simulink model "reactor_2izoterm"  (R2021a)
settings: Solver=VariableStepAuto  StartTime=0.0  StopTime=10.0  RelTol=1e-3
values from neighbouring files (symbols this model uses):
  ci = 10    [script.m]
  EdR = 49584/8.32    (= 5959.61538462)    [script.m]
  k0 = 34930800    [script.m]
  Kr = Tp/(T0int*Kp)    (= 35.3982300885)    [script.m]
  Ti = 38+273    (= 311)    [script.m]
  Tint = Tp    (= 0.78)    [script.m]
  V = 10    [script.m]
libraries: pid_lib x1
settings Model: Creator=Automatica  LastModifiedBy=Automatica

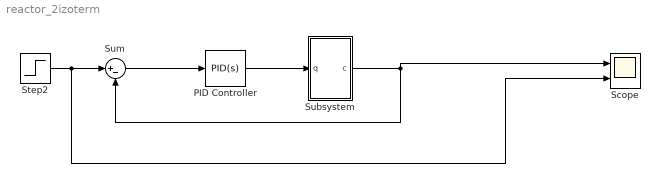
== system reactor_2izoterm ==
  PID Controller : pid_lib/PID Controller  Controller=PID  Form=Parallel  TimeDomain=Continuous-time  UseExternalTs=off  SampleTime=-1  IntegratorMethod=Forward Euler  FilterMethod=Forward Euler  ControllerParametersSource=internal  P=Kr  I=Kr/Tint  D=0  UseFilter=on  N=100  TunerSelectOption=Transfer Function Based (PID Tuner App)  InitialConditionSource=internal  InitialConditionForIntegrator=q  InitialConditionForFilter=0  DifferentiatorICPrevScaledInput=0  ExternalReset=none  TrackingMode=off  Kt=1  LimitOutput=off  SatLimitsSource=internal  UpperSaturationLimit=inf  LowerSaturationLimit=-inf  LinearizeAsGain=on  AntiWindupMode=none  Kb=1  POutMin=[]  POutMax=[]  IOutMin=[]  IOutMax=[]  DOutMin=[]  DOutMax=[]  NOutMin=[]  NOutMax=[]  SumOutMin=[]  SumOutMax=[]  SaturationOutMin=[]  SaturationOutMax=[]  PParamMin=[]  PParamMax=[]  IParamMin=[]  IParamMax=[]  DParamMin=[]  DParamMax=[]  NParamMin=[]  NParamMax=[]  KbParamMin=[]  KbParamMax=[]  KtParamMin=[]  KtParamMax=[]  KbOutMin=[]  KbOutMax=[]  KtOutMin=[]  KtOutMax=[]  IntegratorOutMin=[]  IntegratorOutMax=[]  FilterOutMin=[]  FilterOutMax=[]  SumI1OutMin=[]  SumI1OutMax=[]  SumI2OutMin=[]  SumI2OutMax=[]  SumI3OutMin=[]  SumI3OutMax=[]  SumI4OutMin=[]  SumI4OutMax=[]  SumDOutMin=[]  SumDOutMax=[]  DifferentiatorOutMin=[]  DifferentiatorOutMax=[]  FilterDiffOutCoefMin=[]  FilterDiffOutCoefMax=[]  ReciprocalOutMin=[]  ReciprocalOutMax=[]  SumDenOutMin=[]  SumDenOutMax=[]  SumNumOutMin=[]  SumNumOutMax=[]  DivideOutMin=[]  DivideOutMax=[]  UdiffTsProdOutMin=[]  UdiffTsProdOutMax=[]  NTsProdOutMin=[]  NTsProdOutMax=[]  UintegralTsProdOutMin=[]  UintegralTsProdOutMax=[]  UngainTsProdOutMin=[]  UngainTsProdOutMax=[]  IntegratorContinuousStateAttributes=''  IntegratorStateMustResolveToSignalObject=off  IntegratorRTWStateStorageClass=Auto  FilterContinuousStateAttributes=''  FilterStateMustResolveToSignalObject=off  FilterRTWStateStorageClass=Auto  ParallelPVariant=InternalParameters  IdealPVariant=Disabled  IVariant=InternalParameters  DVariant=InternalParameters  IntegratorVariant=Continuous  SatVariant=Disabled  AWVariant=Passthrough  PCopyVariant=Disabled  TRVariant=Disabled  FdbkBlocksVariant=Forward  IdealPFdbkVariant=Disabled  SatFdbkVariant=Disabled  DerivativeFilterVariant=ContFilter  NVariant=InternalParameters  NCopyVariant=Disabled  FilterICVariant=InternalICsFilter  IntegratorICVariant=InternalICs  ExternalResetVariant=Disabled  TRSumVariant=Passthrough  SumFdbkVariant=Disabled  SumVariant=Sum_PID  TsampFilterVariant=InternalTs  TsampNgainVariant=Passthrough  TsampIntegralVariant=Passthrough  ExternalSaturationOutDataTypeStr=Inherit: Same as second input
  Scope : Scope  NumInputPorts=2
  Step2 : Step  Time=0  Before=8.574  After=8.574+0.1  SampleTime=0
  Subsystem : Subsystem
  Sum : Sum  Inputs=|+-
  wires:
  Subsystem/1(c) -> Sum/2, Scope/1
  Step2/1 -> Scope/2, Sum/1
  PID Controller/1 -> Subsystem/1(q)
  Sum/1 -> PID Controller/1

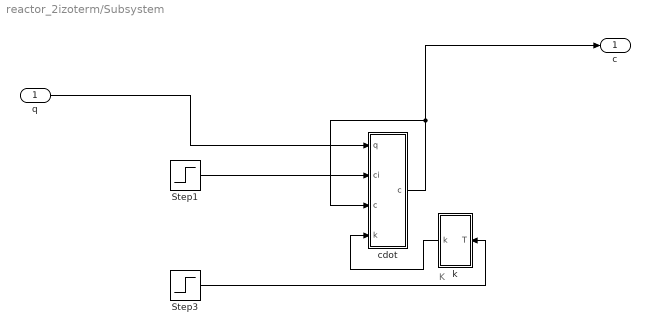
== system reactor_2izoterm/Subsystem ==
  note: K
  q : Inport
  Step1 : Step  Time=0  Before=ci  After=ci  SampleTime=0
  Step3 : Step  Time=0  Before=Ti  After=Ti  SampleTime=0
  cdot : Subsystem
  k : Subsystem
  c : Outport
  wires:
  cdot/1(c) -> c/1, cdot/3("c  ")
  Step3/1 -> k/1(T)
  q/1 -> cdot/1(q)
  Step1/1 -> cdot/2(ci)
  k/1(k) -> cdot/4(k)

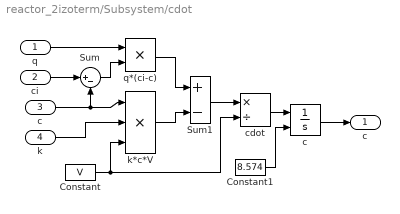
== system reactor_2izoterm/Subsystem/cdot ==
  q : Inport  Interpolate=off
  ci : Inport  Port=2  Interpolate=off
  "c  " : Inport  Port=3  Interpolate=off
  k : Inport  Port=4  Interpolate=off
  Constant : Constant  Value=V
  Constant1 : Constant  Value=8.574
  Sum : Sum  Inputs=|+-  InputSameDT=on  SaturateOnIntegerOverflow=on  OutDataTypeStr=Inherit: Same as first input
  Sum1 : Sum  Inputs=+-  InputSameDT=on  SaturateOnIntegerOverflow=on  OutDataTypeStr=Inherit: Same as first input
  "c " : Integrator  InitialConditionSource=external
  cdot : Product  Inputs=*/  InputSameDT=on  RndMeth=Zero  SaturateOnIntegerOverflow=on  OutDataTypeStr=Inherit: Same as first input
  k*c*V : Product  Inputs=***  InputSameDT=on  RndMeth=Zero  SaturateOnIntegerOverflow=on  OutDataTypeStr=Inherit: Same as first input
  q*(ci-c) : Product  Inputs=**  InputSameDT=on  RndMeth=Zero  SaturateOnIntegerOverflow=on  OutDataTypeStr=Inherit: Same as first input
  c : Outport
  wires:
  ci/1 -> Sum/1
  "c  "/1 -> k*c*V/1, Sum/2
  q/1 -> q*(ci-c)/1
  Sum/1 -> q*(ci-c)/2
  k/1 -> k*c*V/2
  q*(ci-c)/1 -> Sum1/1
  k*c*V/1 -> Sum1/2
  Sum1/1 -> cdot/1
  Constant/1 -> k*c*V/3, cdot/2
  cdot/1 -> "c "/1
  "c "/1 -> c/1
  Constant1/1 -> "c "/2

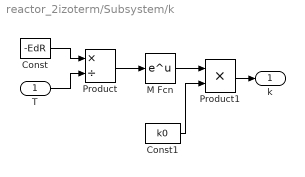
== system reactor_2izoterm/Subsystem/k ==
  T : Inport  Interpolate=off
  Const : Constant  Value=-EdR
  Const1 : Constant  Value=k0
  M Fcn : Math  SignedPower=on  SaturateOnIntegerOverflow=on
  Product : Product  Inputs=*/  InputSameDT=on  RndMeth=Zero  SaturateOnIntegerOverflow=on  OutDataTypeStr=Inherit: Same as first input
  Product1 : Product  Inputs=**  InputSameDT=on  RndMeth=Zero  SaturateOnIntegerOverflow=on  OutDataTypeStr=Inherit: Same as first input
  k : Outport
  wires:
  Const/1 -> Product/1
  T/1 -> Product/2
  Product/1 -> M Fcn/1
  M Fcn/1 -> Product1/1
  Const1/1 -> Product1/2
  Product1/1 -> k/1
